simulink model "carga_suspendida_test"  (R2019a)
settings: Solver=VariableStepAuto  StartTime=0.0  StopTime=10.0  RelTol=1e-3
undefined symbols (not defined in the file): x_t0
libraries: simulink x3
settings Model: Creator=Facundo  LastModifiedBy=Facundo

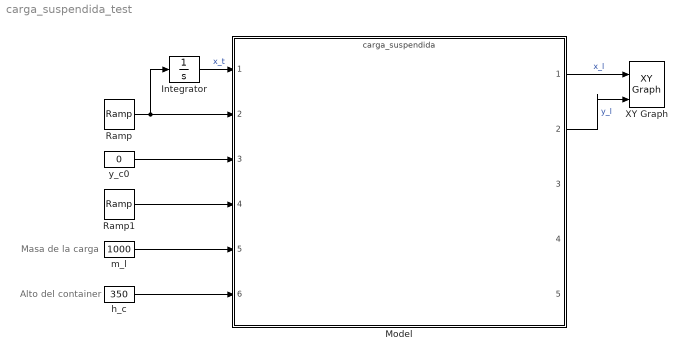
== system carga_suspendida_test ==
  note: Masa de la carga
  note: Alto del container
  Integrator : Integrator  InitialCondition=x_t0
  Model : ModelReference  ModelNameDialog=carga_suspendida.slx  SimulationMode=Normal  ModelReferenceVersion=1.40
  Ramp : simulink/Sources/Ramp  slope=1  start=0.5  InitialOutput=0
  Ramp1 : simulink/Sources/Ramp  slope=20  start=0.5  InitialOutput=0
  XY Graph : simulink/Sinks/XY Graph  xmin=-1000  xmax=1000  ymin=-1000  ymax=1000  st=-1
  h_c : Constant  Value=350
  m_l : Constant  Value=1000
  y_c0 : Constant  Value=0
  wires:
  m_l/1 -> Model/5
  h_c/1 -> Model/6
  Ramp/1 -> Model/2, Integrator/1
  Integrator/1 -> Model/1  "x_t"
  y_c0/1 -> Model/3
  Ramp1/1 -> Model/4
  Model/1 -> XY Graph/1  "x_l"
  Model/2 -> XY Graph/2  "y_l"
